simulink model "dynamiqueLaterale"  (R2021a)
settings: Solver=FixedStepAuto  StartTime=0.0  StopTime=tf_max  FixedStep=ts  RelTol=1e-3
undefined symbols (not defined in the file or in its folder): latdyn, x0
settings Model: Creator=PC_DE_PRET_LDLC  LastModifiedBy=PC_DE_PRET_LDLC

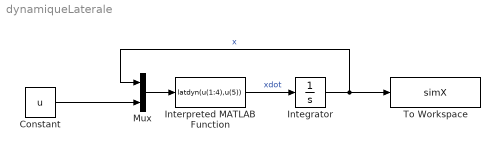
== system dynamiqueLaterale ==
  Constant : Constant  Value=u
  Integrator : Integrator  InitialCondition=x0
  Interpreted MATLAB Function : MATLABFcn  MATLABFcn=latdyn(u(1:4),u(5))
  Mux : Mux  Inputs=2
  To Workspace : ToWorkspace  VariableName=simX  SaveFormat=Timeseries  SampleTime=-1
  wires:
  Mux/1 -> Interpreted MATLAB Function/1
  Interpreted MATLAB Function/1 -> Integrator/1  "xdot"
  Integrator/1 -> To Workspace/1, Mux/1  "x"
  Constant/1 -> Mux/2
